simulink model "IEEE_13_BUS_Radial"  (R2021b)
settings: Solver=VariableStepAuto  StartTime=0.0  StopTime=48  RelTol=1e-3
undefined symbols (not defined in the file or in its folder): f611, f632, f633, f634, f645, f646, f650, f652, f671, f675, f680, f684, f692
libraries: simulink x416, slpidlib x13
(part 1 of 7)
settings Model: Creator=Admin  LastModifiedBy=Admin
settings SolverCC: AlgebraicLoopSolver=TrustRegion
settings DebuggingCC: SFMachineParentedDataDiag=warning

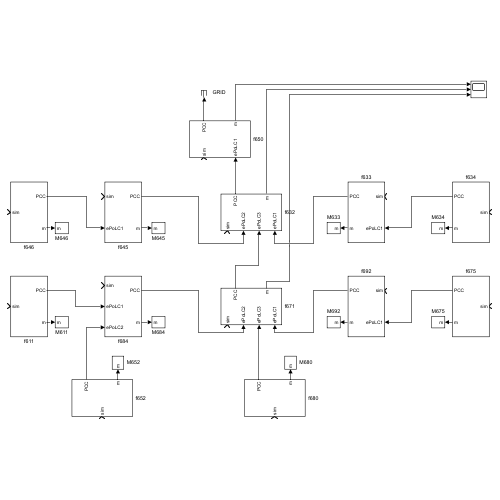
[thumbnail: Simulink's stored preview of the top-level diagram]
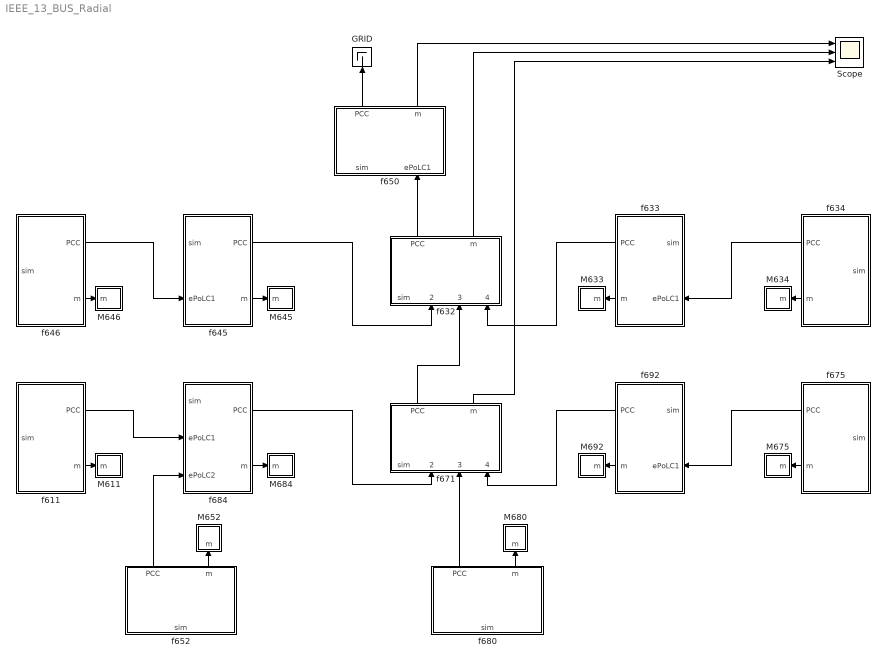
== system IEEE_13_BUS_Radial ==
  GRID : Terminator
  M611 : Subsystem
  M633 : Subsystem
  M634 : Subsystem
  M645 : Subsystem
  M646 : Subsystem
  M652 : Subsystem
  M675 : Subsystem
  M680 : Subsystem
  M684 : Subsystem
  M692 : Subsystem
  Scope : Scope  NumInputPorts=3
  f611 : Subsystem  mask(Prosumer){sPoLC1sel=Internal, sPoLC2sel=Disabled, sPoLC3sel=Disabled, sPoLC4sel=Disabled, sPoLC5sel=Disabled, sPoLC6sel=Disabled, sPoLC7sel=Disabled, sPoLC8sel=Disabled, sPoLC9sel=Disabled, sPoLC10sel=Disabled, sPoLC11sel=Disabled, sPoLC12sel=Disabled, sPoLC13sel=Disabled, sPoLC14sel=Disabled, sPoLC15sel=Disabled, sPoLC16sel=Disabled}
      mask prompts: sPoLC1sel "PoLC #1 type"; sPoLC2sel "PoLC #2 type"; sPoLC3sel "PoLC #3 type"; sPoLC4sel "PoLC #4 type"; sPoLC5sel "PoLC #5 type"; sPoLC6sel "PoLC #6 type"; sPoLC7sel "PoLC #7 type"; sPoLC8sel "PoLC #8 type"; sPoLC9sel "PoLC #9 type"; sPoLC10sel "PoLC #10 type"; sPoLC11sel "PoLC #11 type"; sPoLC12sel "PoLC #12 type"; sPoLC13sel "PoLC #13 type"; sPoLC14sel "PoLC #14 type"; sPoLC15sel "PoLC #15 type"; sPoLC16sel "PoLC #16 type"
      mask help:
      | Simplified model of electrical prosumer technological system.
      |
      | V0.1.0
      mask init:
      | % link local generation variables
      | tblk = Simulink.findBlocks(gcb,'Name','base');
      | for i=1:length(tblk)
      |     val = strrep(getfullname(tblk(i)),join([gcs,'/'],''),'');
      |     val = strrep(val,join(['/','base'],''),'');
      |     val = strrep(val,'lPoLC','PoLC');
      |     val = strrep(val,'DEVICES/','');
      |     val = strrep(val,'CONTROLLERS/','');
      |     val = strrep(val,'/','.');
      |     set_param(tblk(i),'OutValues',join([val,'.','l'],''));
      |     set_param(tblk(i),'tsamp',join([val,'.','ST'],''));
      | end
      | 
      | sblk = Simulink.findBlocks(gcb,'Name','noise');
      | for i=1:length(sblk)
      |     val = strrep(getfullname(sblk(i)),join([gcs,'/'],''),'');
      |     val = strrep(val,join(['/','noise'],''),'');
      |     val = strrep(val,'lPoLC','PoLC');
      |     val = strrep(val,'DEVICES/','');
      |     val = strrep(val,'CONTROLLERS/','');
      |     val = strrep(val,'/','.');
      |     set_param(sblk(i),'Cov',join([val,'.','Noise'],''));
      |     set_param(sblk(i),'Ts',join([val,'.','NoiseST'],''));
      |     set_param(sblk(i),'seed',join([val,'.','NoiseSD'],''));
      | end
      mask TypeOptions sPoLC1sel: Disabled | Internal | External
      mask Callback sPoLC1sel: prsmr_functions('1',gcs,gcb);
      mask TypeOptions sPoLC2sel: Disabled | Internal | External
      mask Callback sPoLC2sel: prsmr_functions('2',gcs,gcb)
      mask TypeOptions sPoLC3sel: Disabled | Internal | External
      mask Callback sPoLC3sel: prsmr_functions('3',gcs,gcb)
      mask TypeOptions sPoLC4sel: Disabled | Internal | External
      mask Callback sPoLC4sel: prsmr_functions('4',gcs,gcb)
      mask TypeOptions sPoLC5sel: Disabled | Internal | External
      mask Callback sPoLC5sel: prsmr_functions('5',gcs,gcb)
      mask TypeOptions sPoLC6sel: Disabled | Internal | External
      mask Callback sPoLC6sel: prsmr_functions('6',gcs,gcb)
      mask TypeOptions sPoLC7sel: Disabled | Internal | External
      mask Callback sPoLC7sel: prsmr_functions('7',gcs,gcb)
      mask TypeOptions sPoLC8sel: Disabled | Internal | External
      mask Callback sPoLC8sel: prsmr_functions('8',gcs,gcb)
      mask TypeOptions sPoLC9sel: Disabled | Internal | External
      mask Callback sPoLC9sel: prsmr_functions('9',gcs,gcb)
      mask TypeOptions sPoLC10sel: Disabled | Internal | External
      mask Callback sPoLC10sel: prsmr_functions('10',gcs,gcb)
      mask TypeOptions sPoLC11sel: Disabled | Internal | External
      mask Callback sPoLC11sel: prsmr_functions('11',gcs,gcb)
      mask TypeOptions sPoLC12sel: Disabled | Internal | External
      mask Callback sPoLC12sel: prsmr_functions('12',gcs,gcb)
      mask TypeOptions sPoLC13sel: Disabled | Internal | External
      mask Callback sPoLC13sel: prsmr_functions('13',gcs,gcb)
      mask TypeOptions sPoLC14sel: Disabled | Internal | External
      mask Callback sPoLC14sel: prsmr_functions('14',gcs,gcb)
      mask TypeOptions sPoLC15sel: Disabled | Internal | External
      mask Callback sPoLC15sel: prsmr_functions('15',gcs,gcb)
      mask TypeOptions sPoLC16sel: Disabled | Internal | External
      mask Callback sPoLC16sel: prsmr_functions('16',gcs,gcb)
  f632 : Subsystem  mask(Prosumer){sPoLC1sel=External, sPoLC2sel=External, sPoLC3sel=External, sPoLC4sel=Disabled, sPoLC5sel=Disabled, sPoLC6sel=Disabled, sPoLC7sel=Disabled, sPoLC8sel=Disabled, sPoLC9sel=Disabled, sPoLC10sel=Disabled, sPoLC11sel=Disabled, sPoLC12sel=Disabled, sPoLC13sel=Disabled, sPoLC14sel=Disabled, sPoLC15sel=Disabled, sPoLC16sel=Disabled}
      mask prompts: sPoLC1sel "PoLC #1 type"; sPoLC2sel "PoLC #2 type"; sPoLC3sel "PoLC #3 type"; sPoLC4sel "PoLC #4 type"; sPoLC5sel "PoLC #5 type"; sPoLC6sel "PoLC #6 type"; sPoLC7sel "PoLC #7 type"; sPoLC8sel "PoLC #8 type"; sPoLC9sel "PoLC #9 type"; sPoLC10sel "PoLC #10 type"; sPoLC11sel "PoLC #11 type"; sPoLC12sel "PoLC #12 type"; sPoLC13sel "PoLC #13 type"; sPoLC14sel "PoLC #14 type"; sPoLC15sel "PoLC #15 type"; sPoLC16sel "PoLC #16 type"
      mask help:
      | Simplified model of electrical prosumer technological system.
      |
      | V0.1.0
      mask init: same as IEEE_13_BUS_Radial/f611
      mask TypeOptions sPoLC1sel: Disabled | Internal | External
      mask Callback sPoLC1sel: prsmr_functions('1',gcs,gcb);
      mask TypeOptions sPoLC2sel: Disabled | Internal | External
      mask Callback sPoLC2sel: prsmr_functions('2',gcs,gcb)
      mask TypeOptions sPoLC3sel: Disabled | Internal | External
      mask Callback sPoLC3sel: prsmr_functions('3',gcs,gcb)
      mask TypeOptions sPoLC4sel: Disabled | Internal | External
      mask Callback sPoLC4sel: prsmr_functions('4',gcs,gcb)
      mask TypeOptions sPoLC5sel: Disabled | Internal | External
      mask Callback sPoLC5sel: prsmr_functions('5',gcs,gcb)
      mask TypeOptions sPoLC6sel: Disabled | Internal | External
      mask Callback sPoLC6sel: prsmr_functions('6',gcs,gcb)
      mask TypeOptions sPoLC7sel: Disabled | Internal | External
      mask Callback sPoLC7sel: prsmr_functions('7',gcs,gcb)
      mask TypeOptions sPoLC8sel: Disabled | Internal | External
      mask Callback sPoLC8sel: prsmr_functions('8',gcs,gcb)
      mask TypeOptions sPoLC9sel: Disabled | Internal | External
      mask Callback sPoLC9sel: prsmr_functions('9',gcs,gcb)
      mask TypeOptions sPoLC10sel: Disabled | Internal | External
      mask Callback sPoLC10sel: prsmr_functions('10',gcs,gcb)
      mask TypeOptions sPoLC11sel: Disabled | Internal | External
      mask Callback sPoLC11sel: prsmr_functions('11',gcs,gcb)
      mask TypeOptions sPoLC12sel: Disabled | Internal | External
      mask Callback sPoLC12sel: prsmr_functions('12',gcs,gcb)
      mask TypeOptions sPoLC13sel: Disabled | Internal | External
      mask Callback sPoLC13sel: prsmr_functions('13',gcs,gcb)
      mask TypeOptions sPoLC14sel: Disabled | Internal | External
      mask Callback sPoLC14sel: prsmr_functions('14',gcs,gcb)
      mask TypeOptions sPoLC15sel: Disabled | Internal | External
      mask Callback sPoLC15sel: prsmr_functions('15',gcs,gcb)
      mask TypeOptions sPoLC16sel: Disabled | Internal | External
      mask Callback sPoLC16sel: prsmr_functions('16',gcs,gcb)
  f633 : Subsystem  mask(Prosumer){sPoLC1sel=External, sPoLC2sel=Disabled, sPoLC3sel=Internal, sPoLC4sel=Disabled, sPoLC5sel=Disabled, sPoLC6sel=Disabled, sPoLC7sel=Disabled, sPoLC8sel=Disabled, sPoLC9sel=Disabled, sPoLC10sel=Disabled, sPoLC11sel=Disabled, sPoLC12sel=Disabled, sPoLC13sel=Disabled, sPoLC14sel=Disabled, sPoLC15sel=Disabled, sPoLC16sel=Disabled}
      mask prompts: sPoLC1sel "PoLC #1 type"; sPoLC2sel "PoLC #2 type"; sPoLC3sel "PoLC #3 type"; sPoLC4sel "PoLC #4 type"; sPoLC5sel "PoLC #5 type"; sPoLC6sel "PoLC #6 type"; sPoLC7sel "PoLC #7 type"; sPoLC8sel "PoLC #8 type"; sPoLC9sel "PoLC #9 type"; sPoLC10sel "PoLC #10 type"; sPoLC11sel "PoLC #11 type"; sPoLC12sel "PoLC #12 type"; sPoLC13sel "PoLC #13 type"; sPoLC14sel "PoLC #14 type"; sPoLC15sel "PoLC #15 type"; sPoLC16sel "PoLC #16 type"
      mask help:
      | Simplified model of electrical prosumer technological system.
      |
      | V0.1.0
      mask init: same as IEEE_13_BUS_Radial/f611
      mask TypeOptions sPoLC1sel: Disabled | Internal | External
      mask Callback sPoLC1sel: prsmr_functions('1',gcs,gcb);
      mask TypeOptions sPoLC2sel: Disabled | Internal | External
      mask Callback sPoLC2sel: prsmr_functions('2',gcs,gcb)
      mask TypeOptions sPoLC3sel: Disabled | Internal | External
      mask Callback sPoLC3sel: prsmr_functions('3',gcs,gcb)
      mask TypeOptions sPoLC4sel: Disabled | Internal | External
      mask Callback sPoLC4sel: prsmr_functions('4',gcs,gcb)
      mask TypeOptions sPoLC5sel: Disabled | Internal | External
      mask Callback sPoLC5sel: prsmr_functions('5',gcs,gcb)
      mask TypeOptions sPoLC6sel: Disabled | Internal | External
      mask Callback sPoLC6sel: prsmr_functions('6',gcs,gcb)
      mask TypeOptions sPoLC7sel: Disabled | Internal | External
      mask Callback sPoLC7sel: prsmr_functions('7',gcs,gcb)
      mask TypeOptions sPoLC8sel: Disabled | Internal | External
      mask Callback sPoLC8sel: prsmr_functions('8',gcs,gcb)
      mask TypeOptions sPoLC9sel: Disabled | Internal | External
      mask Callback sPoLC9sel: prsmr_functions('9',gcs,gcb)
      mask TypeOptions sPoLC10sel: Disabled | Internal | External
      mask Callback sPoLC10sel: prsmr_functions('10',gcs,gcb)
      mask TypeOptions sPoLC11sel: Disabled | Internal | External
      mask Callback sPoLC11sel: prsmr_functions('11',gcs,gcb)
      mask TypeOptions sPoLC12sel: Disabled | Internal | External
      mask Callback sPoLC12sel: prsmr_functions('12',gcs,gcb)
      mask TypeOptions sPoLC13sel: Disabled | Internal | External
      mask Callback sPoLC13sel: prsmr_functions('13',gcs,gcb)
      mask TypeOptions sPoLC14sel: Disabled | Internal | External
      mask Callback sPoLC14sel: prsmr_functions('14',gcs,gcb)
      mask TypeOptions sPoLC15sel: Disabled | Internal | External
      mask Callback sPoLC15sel: prsmr_functions('15',gcs,gcb)
      mask TypeOptions sPoLC16sel: Disabled | Internal | External
      mask Callback sPoLC16sel: prsmr_functions('16',gcs,gcb)
  f634 : Subsystem  mask(Prosumer){sPoLC1sel=Internal, sPoLC2sel=Disabled, sPoLC3sel=Disabled, sPoLC4sel=Disabled, sPoLC5sel=Disabled, sPoLC6sel=Disabled, sPoLC7sel=Disabled, sPoLC8sel=Disabled, sPoLC9sel=Disabled, sPoLC10sel=Disabled, sPoLC11sel=Disabled, sPoLC12sel=Disabled, sPoLC13sel=Disabled, sPoLC14sel=Disabled, sPoLC15sel=Disabled, sPoLC16sel=Disabled}
      mask prompts: sPoLC1sel "PoLC #1 type"; sPoLC2sel "PoLC #2 type"; sPoLC3sel "PoLC #3 type"; sPoLC4sel "PoLC #4 type"; sPoLC5sel "PoLC #5 type"; sPoLC6sel "PoLC #6 type"; sPoLC7sel "PoLC #7 type"; sPoLC8sel "PoLC #8 type"; sPoLC9sel "PoLC #9 type"; sPoLC10sel "PoLC #10 type"; sPoLC11sel "PoLC #11 type"; sPoLC12sel "PoLC #12 type"; sPoLC13sel "PoLC #13 type"; sPoLC14sel "PoLC #14 type"; sPoLC15sel "PoLC #15 type"; sPoLC16sel "PoLC #16 type"
      mask help:
      | Simplified model of electrical prosumer technological system.
      |
      | V0.1.0
      mask init: same as IEEE_13_BUS_Radial/f611
      mask TypeOptions sPoLC1sel: Disabled | Internal | External
      mask Callback sPoLC1sel: prsmr_functions('1',gcs,gcb);
      mask TypeOptions sPoLC2sel: Disabled | Internal | External
      mask Callback sPoLC2sel: prsmr_functions('2',gcs,gcb)
      mask TypeOptions sPoLC3sel: Disabled | Internal | External
      mask Callback sPoLC3sel: prsmr_functions('3',gcs,gcb)
      mask TypeOptions sPoLC4sel: Disabled | Internal | External
      mask Callback sPoLC4sel: prsmr_functions('4',gcs,gcb)
      mask TypeOptions sPoLC5sel: Disabled | Internal | External
      mask Callback sPoLC5sel: prsmr_functions('5',gcs,gcb)
      mask TypeOptions sPoLC6sel: Disabled | Internal | External
      mask Callback sPoLC6sel: prsmr_functions('6',gcs,gcb)
      mask TypeOptions sPoLC7sel: Disabled | Internal | External
      mask Callback sPoLC7sel: prsmr_functions('7',gcs,gcb)
      mask TypeOptions sPoLC8sel: Disabled | Internal | External
      mask Callback sPoLC8sel: prsmr_functions('8',gcs,gcb)
      mask TypeOptions sPoLC9sel: Disabled | Internal | External
      mask Callback sPoLC9sel: prsmr_functions('9',gcs,gcb)
      mask TypeOptions sPoLC10sel: Disabled | Internal | External
      mask Callback sPoLC10sel: prsmr_functions('10',gcs,gcb)
      mask TypeOptions sPoLC11sel: Disabled | Internal | External
      mask Callback sPoLC11sel: prsmr_functions('11',gcs,gcb)
      mask TypeOptions sPoLC12sel: Disabled | Internal | External
      mask Callback sPoLC12sel: prsmr_functions('12',gcs,gcb)
      mask TypeOptions sPoLC13sel: Disabled | Internal | External
      mask Callback sPoLC13sel: prsmr_functions('13',gcs,gcb)
      mask TypeOptions sPoLC14sel: Disabled | Internal | External
      mask Callback sPoLC14sel: prsmr_functions('14',gcs,gcb)
      mask TypeOptions sPoLC15sel: Disabled | Internal | External
      mask Callback sPoLC15sel: prsmr_functions('15',gcs,gcb)
      mask TypeOptions sPoLC16sel: Disabled | Internal | External
      mask Callback sPoLC16sel: prsmr_functions('16',gcs,gcb)
  f645 : Subsystem  mask(Prosumer){sPoLC1sel=External, sPoLC2sel=Internal, sPoLC3sel=Disabled, sPoLC4sel=Disabled, sPoLC5sel=Disabled, sPoLC6sel=Disabled, sPoLC7sel=Disabled, sPoLC8sel=Disabled, sPoLC9sel=Disabled, sPoLC10sel=Disabled, sPoLC11sel=Disabled, sPoLC12sel=Disabled, sPoLC13sel=Disabled, sPoLC14sel=Disabled, sPoLC15sel=Disabled, sPoLC16sel=Disabled}
      mask prompts: sPoLC1sel "PoLC #1 type"; sPoLC2sel "PoLC #2 type"; sPoLC3sel "PoLC #3 type"; sPoLC4sel "PoLC #4 type"; sPoLC5sel "PoLC #5 type"; sPoLC6sel "PoLC #6 type"; sPoLC7sel "PoLC #7 type"; sPoLC8sel "PoLC #8 type"; sPoLC9sel "PoLC #9 type"; sPoLC10sel "PoLC #10 type"; sPoLC11sel "PoLC #11 type"; sPoLC12sel "PoLC #12 type"; sPoLC13sel "PoLC #13 type"; sPoLC14sel "PoLC #14 type"; sPoLC15sel "PoLC #15 type"; sPoLC16sel "PoLC #16 type"
      mask help:
      | Simplified model of electrical prosumer technological system.
      |
      | V0.1.0
      mask init: same as IEEE_13_BUS_Radial/f611
      mask TypeOptions sPoLC1sel: Disabled | Internal | External
      mask Callback sPoLC1sel: prsmr_functions('1',gcs,gcb);
      mask TypeOptions sPoLC2sel: Disabled | Internal | External
      mask Callback sPoLC2sel: prsmr_functions('2',gcs,gcb)
      mask TypeOptions sPoLC3sel: Disabled | Internal | External
      mask Callback sPoLC3sel: prsmr_functions('3',gcs,gcb)
      mask TypeOptions sPoLC4sel: Disabled | Internal | External
      mask Callback sPoLC4sel: prsmr_functions('4',gcs,gcb)
      mask TypeOptions sPoLC5sel: Disabled | Internal | External
      mask Callback sPoLC5sel: prsmr_functions('5',gcs,gcb)
      mask TypeOptions sPoLC6sel: Disabled | Internal | External
      mask Callback sPoLC6sel: prsmr_functions('6',gcs,gcb)
      mask TypeOptions sPoLC7sel: Disabled | Internal | External
      mask Callback sPoLC7sel: prsmr_functions('7',gcs,gcb)
      mask TypeOptions sPoLC8sel: Disabled | Internal | External
      mask Callback sPoLC8sel: prsmr_functions('8',gcs,gcb)
      mask TypeOptions sPoLC9sel: Disabled | Internal | External
      mask Callback sPoLC9sel: prsmr_functions('9',gcs,gcb)
      mask TypeOptions sPoLC10sel: Disabled | Internal | External
      mask Callback sPoLC10sel: prsmr_functions('10',gcs,gcb)
      mask TypeOptions sPoLC11sel: Disabled | Internal | External
      mask Callback sPoLC11sel: prsmr_functions('11',gcs,gcb)
      mask TypeOptions sPoLC12sel: Disabled | Internal | External
      mask Callback sPoLC12sel: prsmr_functions('12',gcs,gcb)
      mask TypeOptions sPoLC13sel: Disabled | Internal | External
      mask Callback sPoLC13sel: prsmr_functions('13',gcs,gcb)
      mask TypeOptions sPoLC14sel: Disabled | Internal | External
      mask Callback sPoLC14sel: prsmr_functions('14',gcs,gcb)
      mask TypeOptions sPoLC15sel: Disabled | Internal | External
      mask Callback sPoLC15sel: prsmr_functions('15',gcs,gcb)
      mask TypeOptions sPoLC16sel: Disabled | Internal | External
      mask Callback sPoLC16sel: prsmr_functions('16',gcs,gcb)
  f646 : Subsystem  mask(Prosumer){sPoLC1sel=Internal, sPoLC2sel=Disabled, sPoLC3sel=Disabled, sPoLC4sel=Disabled, sPoLC5sel=Disabled, sPoLC6sel=Disabled, sPoLC7sel=Disabled, sPoLC8sel=Disabled, sPoLC9sel=Disabled, sPoLC10sel=Disabled, sPoLC11sel=Disabled, sPoLC12sel=Disabled, sPoLC13sel=Disabled, sPoLC14sel=Disabled, sPoLC15sel=Disabled, sPoLC16sel=Disabled}
      mask prompts: sPoLC1sel "PoLC #1 type"; sPoLC2sel "PoLC #2 type"; sPoLC3sel "PoLC #3 type"; sPoLC4sel "PoLC #4 type"; sPoLC5sel "PoLC #5 type"; sPoLC6sel "PoLC #6 type"; sPoLC7sel "PoLC #7 type"; sPoLC8sel "PoLC #8 type"; sPoLC9sel "PoLC #9 type"; sPoLC10sel "PoLC #10 type"; sPoLC11sel "PoLC #11 type"; sPoLC12sel "PoLC #12 type"; sPoLC13sel "PoLC #13 type"; sPoLC14sel "PoLC #14 type"; sPoLC15sel "PoLC #15 type"; sPoLC16sel "PoLC #16 type"
      mask help:
      | Simplified model of electrical prosumer technological system.
      |
      | V0.1.0
      mask init: same as IEEE_13_BUS_Radial/f611
      mask TypeOptions sPoLC1sel: Disabled | Internal | External
      mask Callback sPoLC1sel: prsmr_functions('1',gcs,gcb);
      mask TypeOptions sPoLC2sel: Disabled | Internal | External
      mask Callback sPoLC2sel: prsmr_functions('2',gcs,gcb)
      mask TypeOptions sPoLC3sel: Disabled | Internal | External
      mask Callback sPoLC3sel: prsmr_functions('3',gcs,gcb)
      mask TypeOptions sPoLC4sel: Disabled | Internal | External
      mask Callback sPoLC4sel: prsmr_functions('4',gcs,gcb)
      mask TypeOptions sPoLC5sel: Disabled | Internal | External
      mask Callback sPoLC5sel: prsmr_functions('5',gcs,gcb)
      mask TypeOptions sPoLC6sel: Disabled | Internal | External
      mask Callback sPoLC6sel: prsmr_functions('6',gcs,gcb)
      mask TypeOptions sPoLC7sel: Disabled | Internal | External
      mask Callback sPoLC7sel: prsmr_functions('7',gcs,gcb)
      mask TypeOptions sPoLC8sel: Disabled | Internal | External
      mask Callback sPoLC8sel: prsmr_functions('8',gcs,gcb)
      mask TypeOptions sPoLC9sel: Disabled | Internal | External
      mask Callback sPoLC9sel: prsmr_functions('9',gcs,gcb)
      mask TypeOptions sPoLC10sel: Disabled | Internal | External
      mask Callback sPoLC10sel: prsmr_functions('10',gcs,gcb)
      mask TypeOptions sPoLC11sel: Disabled | Internal | External
      mask Callback sPoLC11sel: prsmr_functions('11',gcs,gcb)
      mask TypeOptions sPoLC12sel: Disabled | Internal | External
      mask Callback sPoLC12sel: prsmr_functions('12',gcs,gcb)
      mask TypeOptions sPoLC13sel: Disabled | Internal | External
      mask Callback sPoLC13sel: prsmr_functions('13',gcs,gcb)
      mask TypeOptions sPoLC14sel: Disabled | Internal | External
      mask Callback sPoLC14sel: prsmr_functions('14',gcs,gcb)
      mask TypeOptions sPoLC15sel: Disabled | Internal | External
      mask Callback sPoLC15sel: prsmr_functions('15',gcs,gcb)
      mask TypeOptions sPoLC16sel: Disabled | Internal | External
      mask Callback sPoLC16sel: prsmr_functions('16',gcs,gcb)
  f650 : Subsystem  mask(Prosumer){sPoLC1sel=External, sPoLC2sel=Disabled, sPoLC3sel=Disabled, sPoLC4sel=Disabled, sPoLC5sel=Disabled, sPoLC6sel=Disabled, sPoLC7sel=Disabled, sPoLC8sel=Disabled, sPoLC9sel=Disabled, sPoLC10sel=Disabled, sPoLC11sel=Disabled, sPoLC12sel=Disabled, sPoLC13sel=Disabled, sPoLC14sel=Disabled, sPoLC15sel=Disabled, sPoLC16sel=Disabled}
      mask prompts: sPoLC1sel "PoLC #1 type"; sPoLC2sel "PoLC #2 type"; sPoLC3sel "PoLC #3 type"; sPoLC4sel "PoLC #4 type"; sPoLC5sel "PoLC #5 type"; sPoLC6sel "PoLC #6 type"; sPoLC7sel "PoLC #7 type"; sPoLC8sel "PoLC #8 type"; sPoLC9sel "PoLC #9 type"; sPoLC10sel "PoLC #10 type"; sPoLC11sel "PoLC #11 type"; sPoLC12sel "PoLC #12 type"; sPoLC13sel "PoLC #13 type"; sPoLC14sel "PoLC #14 type"; sPoLC15sel "PoLC #15 type"; sPoLC16sel "PoLC #16 type"
      mask help:
      | Simplified model of electrical prosumer technological system.
      |
      | V0.1.0
      mask init: same as IEEE_13_BUS_Radial/f611
      mask TypeOptions sPoLC1sel: Disabled | Internal | External
      mask Callback sPoLC1sel: prsmr_functions('1',gcs,gcb);
      mask TypeOptions sPoLC2sel: Disabled | Internal | External
      mask Callback sPoLC2sel: prsmr_functions('2',gcs,gcb)
      mask TypeOptions sPoLC3sel: Disabled | Internal | External
      mask Callback sPoLC3sel: prsmr_functions('3',gcs,gcb)
      mask TypeOptions sPoLC4sel: Disabled | Internal | External
      mask Callback sPoLC4sel: prsmr_functions('4',gcs,gcb)
      mask TypeOptions sPoLC5sel: Disabled | Internal | External
      mask Callback sPoLC5sel: prsmr_functions('5',gcs,gcb)
      mask TypeOptions sPoLC6sel: Disabled | Internal | External
      mask Callback sPoLC6sel: prsmr_functions('6',gcs,gcb)
      mask TypeOptions sPoLC7sel: Disabled | Internal | External
      mask Callback sPoLC7sel: prsmr_functions('7',gcs,gcb)
      mask TypeOptions sPoLC8sel: Disabled | Internal | External
      mask Callback sPoLC8sel: prsmr_functions('8',gcs,gcb)
      mask TypeOptions sPoLC9sel: Disabled | Internal | External
      mask Callback sPoLC9sel: prsmr_functions('9',gcs,gcb)
      mask TypeOptions sPoLC10sel: Disabled | Internal | External
      mask Callback sPoLC10sel: prsmr_functions('10',gcs,gcb)
      mask TypeOptions sPoLC11sel: Disabled | Internal | External
      mask Callback sPoLC11sel: prsmr_functions('11',gcs,gcb)
      mask TypeOptions sPoLC12sel: Disabled | Internal | External
      mask Callback sPoLC12sel: prsmr_functions('12',gcs,gcb)
      mask TypeOptions sPoLC13sel: Disabled | Internal | External
      mask Callback sPoLC13sel: prsmr_functions('13',gcs,gcb)
      mask TypeOptions sPoLC14sel: Disabled | Internal | External
      mask Callback sPoLC14sel: prsmr_functions('14',gcs,gcb)
      mask TypeOptions sPoLC15sel: Disabled | Internal | External
      mask Callback sPoLC15sel: prsmr_functions('15',gcs,gcb)
      mask TypeOptions sPoLC16sel: Disabled | Internal | External
      mask Callback sPoLC16sel: prsmr_functions('16',gcs,gcb)
  f652 : Subsystem  mask(Prosumer){sPoLC1sel=Internal, sPoLC2sel=Disabled, sPoLC3sel=Disabled, sPoLC4sel=Disabled, sPoLC5sel=Disabled, sPoLC6sel=Disabled, sPoLC7sel=Disabled, sPoLC8sel=Disabled, sPoLC9sel=Disabled, sPoLC10sel=Disabled, sPoLC11sel=Disabled, sPoLC12sel=Disabled, sPoLC13sel=Disabled, sPoLC14sel=Disabled, sPoLC15sel=Disabled, sPoLC16sel=Disabled}
      mask prompts: sPoLC1sel "PoLC #1 type"; sPoLC2sel "PoLC #2 type"; sPoLC3sel "PoLC #3 type"; sPoLC4sel "PoLC #4 type"; sPoLC5sel "PoLC #5 type"; sPoLC6sel "PoLC #6 type"; sPoLC7sel "PoLC #7 type"; sPoLC8sel "PoLC #8 type"; sPoLC9sel "PoLC #9 type"; sPoLC10sel "PoLC #10 type"; sPoLC11sel "PoLC #11 type"; sPoLC12sel "PoLC #12 type"; sPoLC13sel "PoLC #13 type"; sPoLC14sel "PoLC #14 type"; sPoLC15sel "PoLC #15 type"; sPoLC16sel "PoLC #16 type"
      mask help:
      | Simplified model of electrical prosumer technological system.
      |
      | V0.1.0
      mask init: same as IEEE_13_BUS_Radial/f611
      mask TypeOptions sPoLC1sel: Disabled | Internal | External
      mask Callback sPoLC1sel: prsmr_functions('1',gcs,gcb);
      mask TypeOptions sPoLC2sel: Disabled | Internal | External
      mask Callback sPoLC2sel: prsmr_functions('2',gcs,gcb)
      mask TypeOptions sPoLC3sel: Disabled | Internal | External
      mask Callback sPoLC3sel: prsmr_functions('3',gcs,gcb)
      mask TypeOptions sPoLC4sel: Disabled | Internal | External
      mask Callback sPoLC4sel: prsmr_functions('4',gcs,gcb)
      mask TypeOptions sPoLC5sel: Disabled | Internal | External
      mask Callback sPoLC5sel: prsmr_functions('5',gcs,gcb)
      mask TypeOptions sPoLC6sel: Disabled | Internal | External
      mask Callback sPoLC6sel: prsmr_functions('6',gcs,gcb)
      mask TypeOptions sPoLC7sel: Disabled | Internal | External
      mask Callback sPoLC7sel: prsmr_functions('7',gcs,gcb)
      mask TypeOptions sPoLC8sel: Disabled | Internal | External
      mask Callback sPoLC8sel: prsmr_functions('8',gcs,gcb)
      mask TypeOptions sPoLC9sel: Disabled | Internal | External
      mask Callback sPoLC9sel: prsmr_functions('9',gcs,gcb)
      mask TypeOptions sPoLC10sel: Disabled | Internal | External
      mask Callback sPoLC10sel: prsmr_functions('10',gcs,gcb)
      mask TypeOptions sPoLC11sel: Disabled | Internal | External
      mask Callback sPoLC11sel: prsmr_functions('11',gcs,gcb)
      mask TypeOptions sPoLC12sel: Disabled | Internal | External
      mask Callback sPoLC12sel: prsmr_functions('12',gcs,gcb)
      mask TypeOptions sPoLC13sel: Disabled | Internal | External
      mask Callback sPoLC13sel: prsmr_functions('13',gcs,gcb)
      mask TypeOptions sPoLC14sel: Disabled | Internal | External
      mask Callback sPoLC14sel: prsmr_functions('14',gcs,gcb)
      mask TypeOptions sPoLC15sel: Disabled | Internal | External
      mask Callback sPoLC15sel: prsmr_functions('15',gcs,gcb)
      mask TypeOptions sPoLC16sel: Disabled | Internal | External
      mask Callback sPoLC16sel: prsmr_functions('16',gcs,gcb)
  f671 : Subsystem  mask(Prosumer){sPoLC1sel=External, sPoLC2sel=External, sPoLC3sel=External, sPoLC4sel=Internal, sPoLC5sel=Internal, sPoLC6sel=Disabled, sPoLC7sel=Disabled, sPoLC8sel=Disabled, sPoLC9sel=Disabled, sPoLC10sel=Disabled, sPoLC11sel=Disabled, sPoLC12sel=Disabled, sPoLC13sel=Disabled, sPoLC14sel=Disabled, sPoLC15sel=Disabled, sPoLC16sel=Disabled}
      mask prompts: sPoLC1sel "PoLC #1 type"; sPoLC2sel "PoLC #2 type"; sPoLC3sel "PoLC #3 type"; sPoLC4sel "PoLC #4 type"; sPoLC5sel "PoLC #5 type"; sPoLC6sel "PoLC #6 type"; sPoLC7sel "PoLC #7 type"; sPoLC8sel "PoLC #8 type"; sPoLC9sel "PoLC #9 type"; sPoLC10sel "PoLC #10 type"; sPoLC11sel "PoLC #11 type"; sPoLC12sel "PoLC #12 type"; sPoLC13sel "PoLC #13 type"; sPoLC14sel "PoLC #14 type"; sPoLC15sel "PoLC #15 type"; sPoLC16sel "PoLC #16 type"
      mask help:
      | Simplified model of electrical prosumer technological system.
      |
      | V0.1.0
      mask init: same as IEEE_13_BUS_Radial/f611
      mask TypeOptions sPoLC1sel: Disabled | Internal | External
      mask Callback sPoLC1sel: prsmr_functions('1',gcs,gcb);
      mask TypeOptions sPoLC2sel: Disabled | Internal | External
      mask Callback sPoLC2sel: prsmr_functions('2',gcs,gcb)
      mask TypeOptions sPoLC3sel: Disabled | Internal | External
      mask Callback sPoLC3sel: prsmr_functions('3',gcs,gcb)
      mask TypeOptions sPoLC4sel: Disabled | Internal | External
      mask Callback sPoLC4sel: prsmr_functions('4',gcs,gcb)
      mask TypeOptions sPoLC5sel: Disabled | Internal | External
      mask Callback sPoLC5sel: prsmr_functions('5',gcs,gcb)
      mask TypeOptions sPoLC6sel: Disabled | Internal | External
      mask Callback sPoLC6sel: prsmr_functions('6',gcs,gcb)
      mask TypeOptions sPoLC7sel: Disabled | Internal | External
      mask Callback sPoLC7sel: prsmr_functions('7',gcs,gcb)
      mask TypeOptions sPoLC8sel: Disabled | Internal | External
      mask Callback sPoLC8sel: prsmr_functions('8',gcs,gcb)
      mask TypeOptions sPoLC9sel: Disabled | Internal | External
      mask Callback sPoLC9sel: prsmr_functions('9',gcs,gcb)
      mask TypeOptions sPoLC10sel: Disabled | Internal | External
      mask Callback sPoLC10sel: prsmr_functions('10',gcs,gcb)
      mask TypeOptions sPoLC11sel: Disabled | Internal | External
      mask Callback sPoLC11sel: prsmr_functions('11',gcs,gcb)
      mask TypeOptions sPoLC12sel: Disabled | Internal | External
      mask Callback sPoLC12sel: prsmr_functions('12',gcs,gcb)
      mask TypeOptions sPoLC13sel: Disabled | Internal | External
      mask Callback sPoLC13sel: prsmr_functions('13',gcs,gcb)
      mask TypeOptions sPoLC14sel: Disabled | Internal | External
      mask Callback sPoLC14sel: prsmr_functions('14',gcs,gcb)
      mask TypeOptions sPoLC15sel: Disabled | Internal | External
      mask Callback sPoLC15sel: prsmr_functions('15',gcs,gcb)
      mask TypeOptions sPoLC16sel: Disabled | Internal | External
      mask Callback sPoLC16sel: prsmr_functions('16',gcs,gcb)
  f675 : Subsystem  mask(Prosumer){sPoLC1sel=Internal, sPoLC2sel=Disabled, sPoLC3sel=Disabled, sPoLC4sel=Disabled, sPoLC5sel=Disabled, sPoLC6sel=Disabled, sPoLC7sel=Disabled, sPoLC8sel=Disabled, sPoLC9sel=Disabled, sPoLC10sel=Disabled, sPoLC11sel=Disabled, sPoLC12sel=Disabled, sPoLC13sel=Disabled, sPoLC14sel=Disabled, sPoLC15sel=Disabled, sPoLC16sel=Disabled}
      mask prompts: sPoLC1sel "PoLC #1 type"; sPoLC2sel "PoLC #2 type"; sPoLC3sel "PoLC #3 type"; sPoLC4sel "PoLC #4 type"; sPoLC5sel "PoLC #5 type"; sPoLC6sel "PoLC #6 type"; sPoLC7sel "PoLC #7 type"; sPoLC8sel "PoLC #8 type"; sPoLC9sel "PoLC #9 type"; sPoLC10sel "PoLC #10 type"; sPoLC11sel "PoLC #11 type"; sPoLC12sel "PoLC #12 type"; sPoLC13sel "PoLC #13 type"; sPoLC14sel "PoLC #14 type"; sPoLC15sel "PoLC #15 type"; sPoLC16sel "PoLC #16 type"
      mask help:
      | Simplified model of electrical prosumer technological system.
      |
      | V0.1.0
      mask init: same as IEEE_13_BUS_Radial/f611
      mask TypeOptions sPoLC1sel: Disabled | Internal | External
      mask Callback sPoLC1sel: prsmr_functions('1',gcs,gcb);
      mask TypeOptions sPoLC2sel: Disabled | Internal | External
      mask Callback sPoLC2sel: prsmr_functions('2',gcs,gcb)
      mask TypeOptions sPoLC3sel: Disabled | Internal | External
      mask Callback sPoLC3sel: prsmr_functions('3',gcs,gcb)
      mask TypeOptions sPoLC4sel: Disabled | Internal | External
      mask Callback sPoLC4sel: prsmr_functions('4',gcs,gcb)
      mask TypeOptions sPoLC5sel: Disabled | Internal | External
      mask Callback sPoLC5sel: prsmr_functions('5',gcs,gcb)
      mask TypeOptions sPoLC6sel: Disabled | Internal | External
      mask Callback sPoLC6sel: prsmr_functions('6',gcs,gcb)
      mask TypeOptions sPoLC7sel: Disabled | Internal | External
      mask Callback sPoLC7sel: prsmr_functions('7',gcs,gcb)
      mask TypeOptions sPoLC8sel: Disabled | Internal | External
      mask Callback sPoLC8sel: prsmr_functions('8',gcs,gcb)
      mask TypeOptions sPoLC9sel: Disabled | Internal | External
      mask Callback sPoLC9sel: prsmr_functions('9',gcs,gcb)
      mask TypeOptions sPoLC10sel: Disabled | Internal | External
      mask Callback sPoLC10sel: prsmr_functions('10',gcs,gcb)
      mask TypeOptions sPoLC11sel: Disabled | Internal | External
      mask Callback sPoLC11sel: prsmr_functions('11',gcs,gcb)
      mask TypeOptions sPoLC12sel: Disabled | Internal | External
      mask Callback sPoLC12sel: prsmr_functions('12',gcs,gcb)
      mask TypeOptions sPoLC13sel: Disabled | Internal | External
      mask Callback sPoLC13sel: prsmr_functions('13',gcs,gcb)
      mask TypeOptions sPoLC14sel: Disabled | Internal | External
      mask Callback sPoLC14sel: prsmr_functions('14',gcs,gcb)
      mask TypeOptions sPoLC15sel: Disabled | Internal | External
      mask Callback sPoLC15sel: prsmr_functions('15',gcs,gcb)
      mask TypeOptions sPoLC16sel: Disabled | Internal | External
      mask Callback sPoLC16sel: prsmr_functions('16',gcs,gcb)
  f680 : Subsystem  mask(Prosumer){sPoLC1sel=Internal, sPoLC2sel=Disabled, sPoLC3sel=Disabled, sPoLC4sel=Disabled, sPoLC5sel=Disabled, sPoLC6sel=Disabled, sPoLC7sel=Disabled, sPoLC8sel=Disabled, sPoLC9sel=Disabled, sPoLC10sel=Disabled, sPoLC11sel=Disabled, sPoLC12sel=Disabled, sPoLC13sel=Disabled, sPoLC14sel=Disabled, sPoLC15sel=Disabled, sPoLC16sel=Disabled}
      mask prompts: sPoLC1sel "PoLC #1 type"; sPoLC2sel "PoLC #2 type"; sPoLC3sel "PoLC #3 type"; sPoLC4sel "PoLC #4 type"; sPoLC5sel "PoLC #5 type"; sPoLC6sel "PoLC #6 type"; sPoLC7sel "PoLC #7 type"; sPoLC8sel "PoLC #8 type"; sPoLC9sel "PoLC #9 type"; sPoLC10sel "PoLC #10 type"; sPoLC11sel "PoLC #11 type"; sPoLC12sel "PoLC #12 type"; sPoLC13sel "PoLC #13 type"; sPoLC14sel "PoLC #14 type"; sPoLC15sel "PoLC #15 type"; sPoLC16sel "PoLC #16 type"
      mask help:
      | Simplified model of electrical prosumer technological system.
      |
      | V0.1.0
      mask init: same as IEEE_13_BUS_Radial/f611
      mask TypeOptions sPoLC1sel: Disabled | Internal | External
      mask Callback sPoLC1sel: prsmr_functions('1',gcs,gcb);
      mask TypeOptions sPoLC2sel: Disabled | Internal | External
      mask Callback sPoLC2sel: prsmr_functions('2',gcs,gcb)
      mask TypeOptions sPoLC3sel: Disabled | Internal | External
      mask Callback sPoLC3sel: prsmr_functions('3',gcs,gcb)
      mask TypeOptions sPoLC4sel: Disabled | Internal | External
      mask Callback sPoLC4sel: prsmr_functions('4',gcs,gcb)
      mask TypeOptions sPoLC5sel: Disabled | Internal | External
      mask Callback sPoLC5sel: prsmr_functions('5',gcs,gcb)
      mask TypeOptions sPoLC6sel: Disabled | Internal | External
      mask Callback sPoLC6sel: prsmr_functions('6',gcs,gcb)
      mask TypeOptions sPoLC7sel: Disabled | Internal | External
      mask Callback sPoLC7sel: prsmr_functions('7',gcs,gcb)
      mask TypeOptions sPoLC8sel: Disabled | Internal | External
      mask Callback sPoLC8sel: prsmr_functions('8',gcs,gcb)
      mask TypeOptions sPoLC9sel: Disabled | Internal | External
      mask Callback sPoLC9sel: prsmr_functions('9',gcs,gcb)
      mask TypeOptions sPoLC10sel: Disabled | Internal | External
      mask Callback sPoLC10sel: prsmr_functions('10',gcs,gcb)
      mask TypeOptions sPoLC11sel: Disabled | Internal | External
      mask Callback sPoLC11sel: prsmr_functions('11',gcs,gcb)
      mask TypeOptions sPoLC12sel: Disabled | Internal | External
      mask Callback sPoLC12sel: prsmr_functions('12',gcs,gcb)
      mask TypeOptions sPoLC13sel: Disabled | Internal | External
      mask Callback sPoLC13sel: prsmr_functions('13',gcs,gcb)
      mask TypeOptions sPoLC14sel: Disabled | Internal | External
      mask Callback sPoLC14sel: prsmr_functions('14',gcs,gcb)
      mask TypeOptions sPoLC15sel: Disabled | Internal | External
      mask Callback sPoLC15sel: prsmr_functions('15',gcs,gcb)
      mask TypeOptions sPoLC16sel: Disabled | Internal | External
      mask Callback sPoLC16sel: prsmr_functions('16',gcs,gcb)
  f684 : Subsystem  mask(Prosumer){sPoLC1sel=External, sPoLC2sel=External, sPoLC3sel=Disabled, sPoLC4sel=Disabled, sPoLC5sel=Disabled, sPoLC6sel=Disabled, sPoLC7sel=Disabled, sPoLC8sel=Disabled, sPoLC9sel=Disabled, sPoLC10sel=Disabled, sPoLC11sel=Disabled, sPoLC12sel=Disabled, sPoLC13sel=Disabled, sPoLC14sel=Disabled, sPoLC15sel=Disabled, sPoLC16sel=Disabled}
      mask prompts: sPoLC1sel "PoLC #1 type"; sPoLC2sel "PoLC #2 type"; sPoLC3sel "PoLC #3 type"; sPoLC4sel "PoLC #4 type"; sPoLC5sel "PoLC #5 type"; sPoLC6sel "PoLC #6 type"; sPoLC7sel "PoLC #7 type"; sPoLC8sel "PoLC #8 type"; sPoLC9sel "PoLC #9 type"; sPoLC10sel "PoLC #10 type"; sPoLC11sel "PoLC #11 type"; sPoLC12sel "PoLC #12 type"; sPoLC13sel "PoLC #13 type"; sPoLC14sel "PoLC #14 type"; sPoLC15sel "PoLC #15 type"; sPoLC16sel "PoLC #16 type"
      mask help:
      | Simplified model of electrical prosumer technological system.
      |
      | V0.1.0
      mask init: same as IEEE_13_BUS_Radial/f611
      mask TypeOptions sPoLC1sel: Disabled | Internal | External
      mask Callback sPoLC1sel: prsmr_functions('1',gcs,gcb);
      mask TypeOptions sPoLC2sel: Disabled | Internal | External
      mask Callback sPoLC2sel: prsmr_functions('2',gcs,gcb)
      mask TypeOptions sPoLC3sel: Disabled | Internal | External
      mask Callback sPoLC3sel: prsmr_functions('3',gcs,gcb)
      mask TypeOptions sPoLC4sel: Disabled | Internal | External
      mask Callback sPoLC4sel: prsmr_functions('4',gcs,gcb)
      mask TypeOptions sPoLC5sel: Disabled | Internal | External
      mask Callback sPoLC5sel: prsmr_functions('5',gcs,gcb)
      mask TypeOptions sPoLC6sel: Disabled | Internal | External
      mask Callback sPoLC6sel: prsmr_functions('6',gcs,gcb)
      mask TypeOptions sPoLC7sel: Disabled | Internal | External
      mask Callback sPoLC7sel: prsmr_functions('7',gcs,gcb)
      mask TypeOptions sPoLC8sel: Disabled | Internal | External
      mask Callback sPoLC8sel: prsmr_functions('8',gcs,gcb)
      mask TypeOptions sPoLC9sel: Disabled | Internal | External
      mask Callback sPoLC9sel: prsmr_functions('9',gcs,gcb)
      mask TypeOptions sPoLC10sel: Disabled | Internal | External
      mask Callback sPoLC10sel: prsmr_functions('10',gcs,gcb)
      mask TypeOptions sPoLC11sel: Disabled | Internal | External
      mask Callback sPoLC11sel: prsmr_functions('11',gcs,gcb)
      mask TypeOptions sPoLC12sel: Disabled | Internal | External
      mask Callback sPoLC12sel: prsmr_functions('12',gcs,gcb)
      mask TypeOptions sPoLC13sel: Disabled | Internal | External
      mask Callback sPoLC13sel: prsmr_functions('13',gcs,gcb)
      mask TypeOptions sPoLC14sel: Disabled | Internal | External
      mask Callback sPoLC14sel: prsmr_functions('14',gcs,gcb)
      mask TypeOptions sPoLC15sel: Disabled | Internal | External
      mask Callback sPoLC15sel: prsmr_functions('15',gcs,gcb)
      mask TypeOptions sPoLC16sel: Disabled | Internal | External
      mask Callback sPoLC16sel: prsmr_functions('16',gcs,gcb)
  f692 : Subsystem  mask(Prosumer){sPoLC1sel=External, sPoLC2sel=Internal, sPoLC3sel=Disabled, sPoLC4sel=Disabled, sPoLC5sel=Disabled, sPoLC6sel=Disabled, sPoLC7sel=Disabled, sPoLC8sel=Disabled, sPoLC9sel=Disabled, sPoLC10sel=Disabled, sPoLC11sel=Disabled, sPoLC12sel=Disabled, sPoLC13sel=Disabled, sPoLC14sel=Disabled, sPoLC15sel=Disabled, sPoLC16sel=Disabled}
      mask prompts: sPoLC1sel "PoLC #1 type"; sPoLC2sel "PoLC #2 type"; sPoLC3sel "PoLC #3 type"; sPoLC4sel "PoLC #4 type"; sPoLC5sel "PoLC #5 type"; sPoLC6sel "PoLC #6 type"; sPoLC7sel "PoLC #7 type"; sPoLC8sel "PoLC #8 type"; sPoLC9sel "PoLC #9 type"; sPoLC10sel "PoLC #10 type"; sPoLC11sel "PoLC #11 type"; sPoLC12sel "PoLC #12 type"; sPoLC13sel "PoLC #13 type"; sPoLC14sel "PoLC #14 type"; sPoLC15sel "PoLC #15 type"; sPoLC16sel "PoLC #16 type"
      mask help:
      | Simplified model of electrical prosumer technological system.
      |
      | V0.1.0
      mask init: same as IEEE_13_BUS_Radial/f611
      mask TypeOptions sPoLC1sel: Disabled | Internal | External
      mask Callback sPoLC1sel: prsmr_functions('1',gcs,gcb);
      mask TypeOptions sPoLC2sel: Disabled | Internal | External
      mask Callback sPoLC2sel: prsmr_functions('2',gcs,gcb)
      mask TypeOptions sPoLC3sel: Disabled | Internal | External
      mask Callback sPoLC3sel: prsmr_functions('3',gcs,gcb)
      mask TypeOptions sPoLC4sel: Disabled | Internal | External
      mask Callback sPoLC4sel: prsmr_functions('4',gcs,gcb)
      mask TypeOptions sPoLC5sel: Disabled | Internal | External
      mask Callback sPoLC5sel: prsmr_functions('5',gcs,gcb)
      mask TypeOptions sPoLC6sel: Disabled | Internal | External
      mask Callback sPoLC6sel: prsmr_functions('6',gcs,gcb)
      mask TypeOptions sPoLC7sel: Disabled | Internal | External
      mask Callback sPoLC7sel: prsmr_functions('7',gcs,gcb)
      mask TypeOptions sPoLC8sel: Disabled | Internal | External
      mask Callback sPoLC8sel: prsmr_functions('8',gcs,gcb)
      mask TypeOptions sPoLC9sel: Disabled | Internal | External
      mask Callback sPoLC9sel: prsmr_functions('9',gcs,gcb)
      mask TypeOptions sPoLC10sel: Disabled | Internal | External
      mask Callback sPoLC10sel: prsmr_functions('10',gcs,gcb)
      mask TypeOptions sPoLC11sel: Disabled | Internal | External
      mask Callback sPoLC11sel: prsmr_functions('11',gcs,gcb)
      mask TypeOptions sPoLC12sel: Disabled | Internal | External
      mask Callback sPoLC12sel: prsmr_functions('12',gcs,gcb)
      mask TypeOptions sPoLC13sel: Disabled | Internal | External
      mask Callback sPoLC13sel: prsmr_functions('13',gcs,gcb)
      mask TypeOptions sPoLC14sel: Disabled | Internal | External
      mask Callback sPoLC14sel: prsmr_functions('14',gcs,gcb)
      mask TypeOptions sPoLC15sel: Disabled | Internal | External
      mask Callback sPoLC15sel: prsmr_functions('15',gcs,gcb)
      mask TypeOptions sPoLC16sel: Disabled | Internal | External
      mask Callback sPoLC16sel: prsmr_functions('16',gcs,gcb)
  wires:
  f650/2(m) -> Scope/1
  f650/1(PCC) -> GRID/1
  f646/1(PCC) -> f645/2(ePoLC1)
  f634/1(PCC) -> f633/2(ePoLC1)
  f633/1(PCC) -> f632/4(ePoLC1)
  f632/1(PCC) -> f650/2(ePoLC1)
  f645/1(PCC) -> f632/2(ePoLC2)
  f675/1(PCC) -> f692/2(ePoLC1)
  f692/1(PCC) -> f671/4(ePoLC1)
  f684/1(PCC) -> f671/2(ePoLC2)
  f611/1(PCC) -> f684/2(ePoLC1)
  f652/1(PCC) -> f684/3(ePoLC2)
  f680/1(PCC) -> f671/3(ePoLC3)
  f671/1(PCC) -> f632/3(ePoLC3)
  f632/2(m) -> Scope/2
  f671/2(m) -> Scope/3
  f646/2(m) -> M646/1(m)
  f645/2(m) -> M645/1(m)
  f611/2(m) -> M611/1(m)
  f684/2(m) -> M684/1(m)
  f652/2(m) -> M652/1(m)
  f680/2(m) -> M680/1(m)
  f692/2(m) -> M692/1(m)
  f675/2(m) -> M675/1(m)
  f634/2(m) -> M634/1(m)
  f633/2(m) -> M633/1(m)

== system IEEE_13_BUS_Radial/M611 ==
  m : Inport
  M611 : Scope
  wires:
  m/1 -> M611/1

== system IEEE_13_BUS_Radial/M633 ==
  m : Inport
  M633 : Scope
  wires:
  m/1 -> M633/1

== system IEEE_13_BUS_Radial/M634 ==
  m : Inport
  M634 : Scope
  wires:
  m/1 -> M634/1

== system IEEE_13_BUS_Radial/M645 ==
  m : Inport
  M645 : Scope
  wires:
  m/1 -> M645/1

== system IEEE_13_BUS_Radial/M646 ==
  m : Inport
  M646 : Scope
  wires:
  m/1 -> M646/1

== system IEEE_13_BUS_Radial/M652 ==
  m : Inport
  M652 : Scope
  wires:
  m/1 -> M652/1

== system IEEE_13_BUS_Radial/M675 ==
  m : Inport
  M675 : Scope
  wires:
  m/1 -> M675/1

== system IEEE_13_BUS_Radial/M680 ==
  m : Inport
  M680 : Scope
  wires:
  m/1 -> M680/1

== system IEEE_13_BUS_Radial/M684 ==
  m : Inport
  M684 : Scope
  wires:
  m/1 -> M684/1

== system IEEE_13_BUS_Radial/M692 ==
  m : Inport
  M692 : Scope
  wires:
  m/1 -> M692/1

== system IEEE_13_BUS_Radial/f611 ==
  note: PROCESS
  note: STATION
  note: FIELD
  note: DISTRIBUTION
  note: CUSTOMER PREMISE & DER
  sim : Inport
  Add : Sum  Inputs=16
  CONTROLLERS : Subsystem
  DEVICES : Subsystem
  Island : Constant  Value=0
  Mux : Mux  Inputs=3
  Mux1 : Mux  Inputs=16
  OPERATIONS GATEWAY : Subsystem
  PCU : Subsystem
  S PCC : Switch  Criteria=u2 > Threshold
  SYSTEM_INTERFACE : Subsystem
  ePoLC{1..16} (16 alike) : Constant  Value=0
  PCC : Outport  VectorParamsAs1DForOutWhenUnconnected=off
  m : Outport  Port=2  VectorParamsAs1DForOutWhenUnconnected=off
  wires:
  PCU/1(PCCctrl) -> S PCC/2
  Mux1/1 -> Mux/2
  Island/1 -> S PCC/1
  Mux/1 -> CONTROLLERS/2(m), PCU/1(m), m/1
  S PCC/1 -> Mux/1, PCC/1
  Add/1 -> S PCC/3
  SYSTEM_INTERFACE/2(PoLC2) -> Add/2, Mux1/2
  SYSTEM_INTERFACE/4(PoLC4) -> Add/4, Mux1/4
  SYSTEM_INTERFACE/8(PoLC8) -> Add/8, Mux1/8
  SYSTEM_INTERFACE/5(PoLC5) -> Add/5, Mux1/5
  SYSTEM_INTERFACE/12(PoLC12) -> Add/12, Mux1/12
  SYSTEM_INTERFACE/15(PoLC15) -> Mux1/15, Add/15
  SYSTEM_INTERFACE/6(PoLC6) -> Add/6, Mux1/6
  SYSTEM_INTERFACE/13(PoLC13) -> Add/13, Mux1/13
  SYSTEM_INTERFACE/10(PoLC10) -> Mux1/10, Add/10
  SYSTEM_INTERFACE/3(PoLC3) -> Add/3, Mux1/3
  SYSTEM_INTERFACE/16(PoLC16) -> Add/16, Mux1/16
  SYSTEM_INTERFACE/1(PoLC1) -> Add/1, Mux1/1
  SYSTEM_INTERFACE/11(PoLC11) -> Add/11, Mux1/11
  SYSTEM_INTERFACE/9(PoLC9) -> Add/9, Mux1/9
  SYSTEM_INTERFACE/7(PoLC7) -> Add/7, Mux1/7
  SYSTEM_INTERFACE/14(PoLC14) -> Add/14, Mux1/14
  ePoLC1/1 -> SYSTEM_INTERFACE/3(e_PoLC1)
  ePoLC2/1 -> SYSTEM_INTERFACE/4(e_PoLC2)
  ePoLC3/1 -> SYSTEM_INTERFACE/5(e_PoLC3)
  ePoLC4/1 -> SYSTEM_INTERFACE/6(e_PoLC4)
  ePoLC5/1 -> SYSTEM_INTERFACE/7(e_PoLC5)
  ePoLC6/1 -> SYSTEM_INTERFACE/8(e_PoLC6)
  ePoLC7/1 -> SYSTEM_INTERFACE/9(e_PoLC7)
  ePoLC8/1 -> SYSTEM_INTERFACE/10(e_PoLC8)
  ePoLC9/1 -> SYSTEM_INTERFACE/11(e_PoLC9)
  ePoLC10/1 -> SYSTEM_INTERFACE/12(e_PoLC10)
  ePoLC11/1 -> SYSTEM_INTERFACE/13(e_PoLC11)
  ePoLC12/1 -> SYSTEM_INTERFACE/14(e_PoLC12)
  ePoLC13/1 -> SYSTEM_INTERFACE/15(e_PoLC13)
  ePoLC14/1 -> SYSTEM_INTERFACE/16(e_PoLC14)
  ePoLC15/1 -> SYSTEM_INTERFACE/17(e_PoLC15)
  ePoLC16/1 -> SYSTEM_INTERFACE/18(e_PoLC16)
  PCU/2(PoLCctrl) -> SYSTEM_INTERFACE/1(ctrl)
  CONTROLLERS/1(dev) -> DEVICES/1(ctrl)
  OPERATIONS GATEWAY/1(setup) -> PCU/2(setup)
  OPERATIONS GATEWAY/2(Psp) -> Mux/3, PCU/3(Psp)
  sim/1 -> OPERATIONS GATEWAY/1(sim)
  PCU/3(DEVctrl) -> CONTROLLERS/1(ctrl)
  DEVICES/1(dev) -> SYSTEM_INTERFACE/2(devices)

== system IEEE_13_BUS_Radial/f632 ==
  note: CUSTOMER PREMISE & DER
  note: DISTRIBUTION
  note: FIELD
  note: STATION
  note: PROCESS
  sim : Inport
  ePoLC2 : Inport  Port=2
  ePoLC3 : Inport  Port=3
  ePoLC1 : Inport  Port=4
  Add : Sum  Inputs=16
  CONTROLLERS : Subsystem
  DEVICES : Subsystem
  Island : Constant  Value=0
  Mux : Mux  Inputs=3
  Mux1 : Mux  Inputs=16
  OPERATIONS GATEWAY : Subsystem
  PCU : Subsystem
  S PCC : Switch  Criteria=u2 > Threshold
  SYSTEM_INTERFACE : Subsystem
  ePoLC{4..16} (13 alike) : Constant  Value=0
  PCC : Outport  VectorParamsAs1DForOutWhenUnconnected=off
  m : Outport  Port=2  VectorParamsAs1DForOutWhenUnconnected=off
  wires:
  DEVICES/1(dev) -> SYSTEM_INTERFACE/2(devices)
  PCU/3(DEVctrl) -> CONTROLLERS/1(ctrl)
  sim/1 -> OPERATIONS GATEWAY/1(sim)
  OPERATIONS GATEWAY/2(Psp) -> PCU/3(Psp), Mux/3
  OPERATIONS GATEWAY/1(setup) -> PCU/2(setup)
  CONTROLLERS/1(dev) -> DEVICES/1(ctrl)
  PCU/2(PoLCctrl) -> SYSTEM_INTERFACE/1(ctrl)
  ePoLC16/1 -> SYSTEM_INTERFACE/18(e_PoLC16)
  ePoLC15/1 -> SYSTEM_INTERFACE/17(e_PoLC15)
  ePoLC14/1 -> SYSTEM_INTERFACE/16(e_PoLC14)
  ePoLC13/1 -> SYSTEM_INTERFACE/15(e_PoLC13)
  ePoLC12/1 -> SYSTEM_INTERFACE/14(e_PoLC12)
  ePoLC11/1 -> SYSTEM_INTERFACE/13(e_PoLC11)
  ePoLC10/1 -> SYSTEM_INTERFACE/12(e_PoLC10)
  ePoLC9/1 -> SYSTEM_INTERFACE/11(e_PoLC9)
  ePoLC8/1 -> SYSTEM_INTERFACE/10(e_PoLC8)
  ePoLC7/1 -> SYSTEM_INTERFACE/9(e_PoLC7)
  ePoLC6/1 -> SYSTEM_INTERFACE/8(e_PoLC6)
  ePoLC5/1 -> SYSTEM_INTERFACE/7(e_PoLC5)
  ePoLC4/1 -> SYSTEM_INTERFACE/6(e_PoLC4)
  ePoLC3/1 -> SYSTEM_INTERFACE/5(e_PoLC3)
  ePoLC2/1 -> SYSTEM_INTERFACE/4(e_PoLC2)
  ePoLC1/1 -> SYSTEM_INTERFACE/3(e_PoLC1)
  SYSTEM_INTERFACE/14(PoLC14) -> Mux1/14, Add/14
  SYSTEM_INTERFACE/7(PoLC7) -> Mux1/7, Add/7
  SYSTEM_INTERFACE/9(PoLC9) -> Mux1/9, Add/9
  SYSTEM_INTERFACE/11(PoLC11) -> Mux1/11, Add/11
  SYSTEM_INTERFACE/1(PoLC1) -> Mux1/1, Add/1
  SYSTEM_INTERFACE/16(PoLC16) -> Mux1/16, Add/16
  SYSTEM_INTERFACE/3(PoLC3) -> Mux1/3, Add/3
  SYSTEM_INTERFACE/10(PoLC10) -> Add/10, Mux1/10
  SYSTEM_INTERFACE/13(PoLC13) -> Mux1/13, Add/13
  SYSTEM_INTERFACE/6(PoLC6) -> Mux1/6, Add/6
  SYSTEM_INTERFACE/15(PoLC15) -> Add/15, Mux1/15
  SYSTEM_INTERFACE/12(PoLC12) -> Mux1/12, Add/12
  SYSTEM_INTERFACE/5(PoLC5) -> Mux1/5, Add/5
  SYSTEM_INTERFACE/8(PoLC8) -> Mux1/8, Add/8
  SYSTEM_INTERFACE/4(PoLC4) -> Mux1/4, Add/4
  SYSTEM_INTERFACE/2(PoLC2) -> Mux1/2, Add/2
  Add/1 -> S PCC/3
  S PCC/1 -> PCC/1, Mux/1
  Mux/1 -> m/1, PCU/1(m), CONTROLLERS/2(m)
  Island/1 -> S PCC/1
  Mux1/1 -> Mux/2
  PCU/1(PCCctrl) -> S PCC/2

== system IEEE_13_BUS_Radial/f633 ==
  note: PROCESS
  note: STATION
  note: FIELD
  note: DISTRIBUTION
  note: CUSTOMER PREMISE & DER
  sim : Inport
  ePoLC1 : Inport  Port=2
  Add : Sum  Inputs=16
  CONTROLLERS : Subsystem
  DEVICES : Subsystem
  Island : Constant  Value=0
  Mux : Mux  Inputs=3
  Mux1 : Mux  Inputs=16
  OPERATIONS GATEWAY : Subsystem
  PCU : Subsystem
  S PCC : Switch  Criteria=u2 > Threshold
  SYSTEM_INTERFACE : Subsystem
  ePoLC{2..16} (15 alike) : Constant  Value=0
  PCC : Outport  VectorParamsAs1DForOutWhenUnconnected=off
  m : Outport  Port=2  VectorParamsAs1DForOutWhenUnconnected=off
  wires:
  PCU/1(PCCctrl) -> S PCC/2
  Mux1/1 -> Mux/2
  Island/1 -> S PCC/1
  Mux/1 -> CONTROLLERS/2(m), PCU/1(m), m/1
  S PCC/1 -> Mux/1, PCC/1
  Add/1 -> S PCC/3
  SYSTEM_INTERFACE/2(PoLC2) -> Add/2, Mux1/2
  SYSTEM_INTERFACE/4(PoLC4) -> Add/4, Mux1/4
  SYSTEM_INTERFACE/8(PoLC8) -> Add/8, Mux1/8
  SYSTEM_INTERFACE/5(PoLC5) -> Add/5, Mux1/5
  SYSTEM_INTERFACE/12(PoLC12) -> Add/12, Mux1/12
  SYSTEM_INTERFACE/15(PoLC15) -> Mux1/15, Add/15
  SYSTEM_INTERFACE/6(PoLC6) -> Add/6, Mux1/6
  SYSTEM_INTERFACE/13(PoLC13) -> Add/13, Mux1/13
  SYSTEM_INTERFACE/10(PoLC10) -> Mux1/10, Add/10
  SYSTEM_INTERFACE/3(PoLC3) -> Add/3, Mux1/3
  SYSTEM_INTERFACE/16(PoLC16) -> Add/16, Mux1/16
  SYSTEM_INTERFACE/1(PoLC1) -> Add/1, Mux1/1
  SYSTEM_INTERFACE/11(PoLC11) -> Add/11, Mux1/11
  SYSTEM_INTERFACE/9(PoLC9) -> Add/9, Mux1/9
  SYSTEM_INTERFACE/7(PoLC7) -> Add/7, Mux1/7
  SYSTEM_INTERFACE/14(PoLC14) -> Add/14, Mux1/14
  ePoLC1/1 -> SYSTEM_INTERFACE/3(e_PoLC1)
  ePoLC2/1 -> SYSTEM_INTERFACE/4(e_PoLC2)
  ePoLC3/1 -> SYSTEM_INTERFACE/5(e_PoLC3)
  ePoLC4/1 -> SYSTEM_INTERFACE/6(e_PoLC4)
  ePoLC5/1 -> SYSTEM_INTERFACE/7(e_PoLC5)
  ePoLC6/1 -> SYSTEM_INTERFACE/8(e_PoLC6)
  ePoLC7/1 -> SYSTEM_INTERFACE/9(e_PoLC7)
  ePoLC8/1 -> SYSTEM_INTERFACE/10(e_PoLC8)
  ePoLC9/1 -> SYSTEM_INTERFACE/11(e_PoLC9)
  ePoLC10/1 -> SYSTEM_INTERFACE/12(e_PoLC10)
  ePoLC11/1 -> SYSTEM_INTERFACE/13(e_PoLC11)
  ePoLC12/1 -> SYSTEM_INTERFACE/14(e_PoLC12)
  ePoLC13/1 -> SYSTEM_INTERFACE/15(e_PoLC13)
  ePoLC14/1 -> SYSTEM_INTERFACE/16(e_PoLC14)
  ePoLC15/1 -> SYSTEM_INTERFACE/17(e_PoLC15)
  ePoLC16/1 -> SYSTEM_INTERFACE/18(e_PoLC16)
  PCU/2(PoLCctrl) -> SYSTEM_INTERFACE/1(ctrl)
  CONTROLLERS/1(dev) -> DEVICES/1(ctrl)
  OPERATIONS GATEWAY/1(setup) -> PCU/2(setup)
  OPERATIONS GATEWAY/2(Psp) -> Mux/3, PCU/3(Psp)
  sim/1 -> OPERATIONS GATEWAY/1(sim)
  PCU/3(DEVctrl) -> CONTROLLERS/1(ctrl)
  DEVICES/1(dev) -> SYSTEM_INTERFACE/2(devices)
